simulink model "mass_spring5"  (R2022b)
settings: Solver=VariableStepAuto  StartTime=0.0  StopTime=Sim_Tim  RelTol=1e-3
undefined symbols (not defined in the file): b, F, k, m
settings Model: Creator=HashimAbdulAzizHashi  LastModifiedBy=HashimAbdulAzizHashi

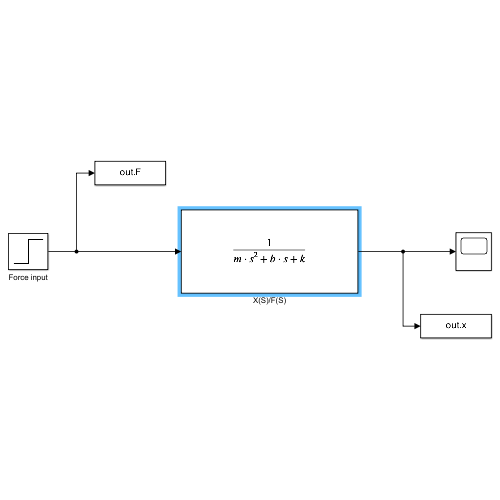
[thumbnail: Simulink's stored preview of the top-level diagram]
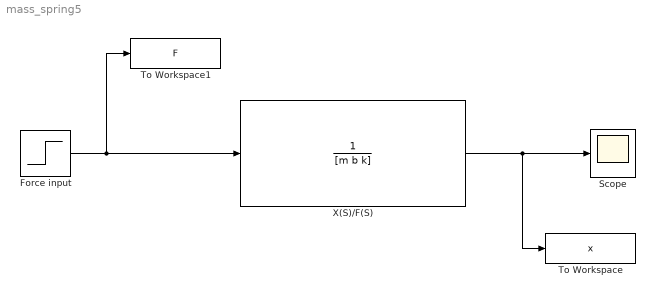
== system mass_spring5 ==
  Force input : Step  After=F  SampleTime=0
  Scope : Scope
  To Workspace : ToWorkspace  VariableName=x  SaveFormat=Timeseries  SampleTime=-1
  To Workspace1 : ToWorkspace  VariableName=F  SaveFormat=Timeseries  SampleTime=-1
  X(S)/F(S) : TransferFcn  Denominator=[m b k]
  wires:
  Force input/1 -> X(S)/F(S)/1, To Workspace1/1
  X(S)/F(S)/1 -> To Workspace/1, Scope/1
